simulink model "SimulinkBATproject"  (R2022b)
settings: Solver=FixedStepAuto  StartTime=0.0  StopTime=15  FixedStep=1e-4  RelTol=1e-3
libraries: spsDiodeLib x12, spsPVArrayLib x10, spsSeriesRLCBranchLib x5, spsCurrentMeasurementLib x1, spsMosfetLib x1, spsPWMGeneratorDCDCLib x1, spsVoltageMeasurementLib x1, spspowerguiLib x1
settings Model: Creator=ACER  LastModifiedBy=LE QUOC DINH
settings SolverCC: AlgebraicLoopSolver=TrustRegion
settings DataIOCC: ReturnWorkspaceOutputs=off
settings DebuggingCC: UnconnectedInputMsg=warning  UnconnectedOutputMsg=warning  UnconnectedLineMsg=warning  PregeneratedLibrarySubsystemCodeDiagnostic=none  SFMachineParentedDataDiag=warning  ArithmeticOperatorsInVariantConditions=warning
settings ModelReferenceCC: EnableRefExpFcnMdlSchedulingChecks=on
settings SFSimCC: SimUseLocalCustomCode=off  CustomCodeUndefinedFunction=UseInterfaceOnly
settings RTWCC: RTWUseLocalCustomCode=off

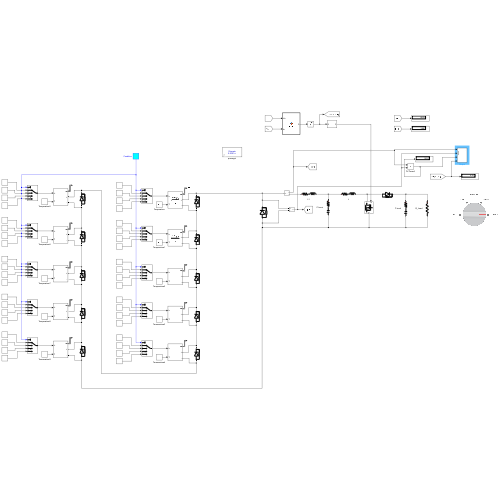
[thumbnail: Simulink's stored preview of the top-level diagram]
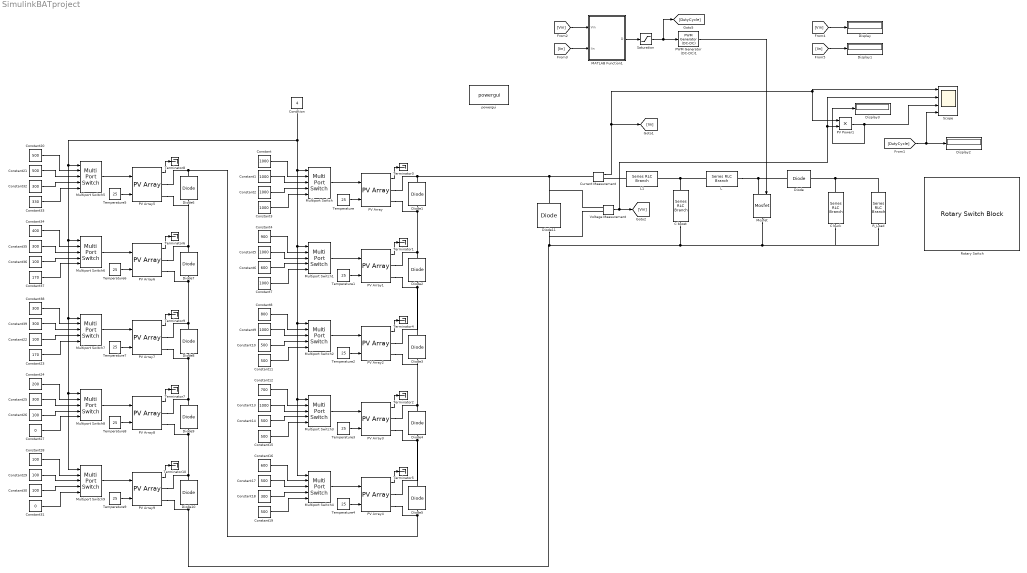
== system SimulinkBATproject ==
  C boost : spsSeriesRLCBranchLib/Series RLC Branch  LConnTagsString=__new0  RConnTagsString=__new0  BranchType=RC  Resistance=1  Inductance=1e-3  SetiL0=off  InitialCurrent=0  Capacitance=50e-3  Setx0=off  InitialVoltage=0  Measurements=None
  C buck : spsSeriesRLCBranchLib/Series RLC Branch  LConnTagsString=__new0  RConnTagsString=__new0  BranchType=RC  Resistance=1  Inductance=1e-3  SetiL0=off  InitialCurrent=0  Capacitance=150e-6  Setx0=off  InitialVoltage=0  Measurements=None
  Condition : Constant  Value=4
  Constant{,1..3,5,7,9,13} (8 alike) : Constant  Value=1000
  Constant{10..11,14..15,17,19..21} (8 alike) : Constant  Value=500
  Constant12 : Constant  Value=700
  Constant16 : Constant  Value=600
  Constant{18,25,32,35,38..39} (6 alike) : Constant  Value=300
  Constant{22,26,28..30,36} (6 alike) : Constant  Value=100
  Constant23 : Constant  Value=170
  Constant24 : Constant  Value=200
  Constant27 : Constant  Value=0
  Constant31 : Constant  Value=0
  Constant33 : Constant  Value=330
  Constant34 : Constant  Value=400
  Constant37 : Constant  Value=170
  Constant4 : Constant  Value=900
  Constant6 : Constant  Value=600
  Constant8 : Constant  Value=800
  Current Measurement : spsCurrentMeasurementLib/Current Measurement  PhasorSimulation=off  OutputType=Complex  PSBequivalent=0
  Diode{,1..11} (12 alike) : spsDiodeLib/Diode  Ron=0.001  Lon=0  Vf=0.8  IC=0  UseSnubber=0  Rs=500  Cs=250e-9  Measurements=off
  Display{,1..3} (4 alike) : Display
  L : spsSeriesRLCBranchLib/Series RLC Branch  LConnTagsString=__new0  RConnTagsString=__new0  BranchType=RL  Resistance=1  Inductance=100e-3  SetiL0=off  InitialCurrent=0  Capacitance=1e-6  Setx0=off  InitialVoltage=0  Measurements=None
  L1 : spsSeriesRLCBranchLib/Series RLC Branch  LConnTagsString=__new0  RConnTagsString=__new0  BranchType=RL  Resistance=1  Inductance=100e-3  SetiL0=off  InitialCurrent=0  Capacitance=1e-6  Setx0=off  InitialVoltage=0  Measurements=None
  MATLAB Function1 : MATLAB Function  TreatAsAtomicUnit=on
  Mosfet : spsMosfetLib/Mosfet  Ron=0.1  Lon=0  Rd=0.01  Vfd=0  IC=0  Rs=1e5  Cs=inf  Measurements=off
  Multiport Switch{,1..9} (10 alike) : MultiPortSwitch  Inputs=4  SaturateOnIntegerOverflow=off  InputSameDT=off
  PV Array{,1..9} (10 alike) : spsPVArrayLib/PV Array  Npar=1  Nser=1  PlotType=array @ 25 deg.C & specified irradiances  S_vec="[ 1000  500  100 ]"  Temp_C_vec="[ 45 25  ]"  ModuleName=Mitsubishi Electric PV-EE125MF5F  PlotWhenSelected=off  Pm=125.079  Ncell=36  Voc=21.8  Isc=7.9  Vm=17.3  Im=7.23  beta_Voc_pc=-0.3637  alpha_Isc_pc=0.042696  beta_Voc=-0.079287  alpha_Isc=0.003373  IL=7.9305  I0=2.9341e-10  nI=0.98298  Rsh=66.3188  Rs=0.25575  RobustModel=off  RobustCellTemperature=313.3991  BAL=off  Tc=20  Tfilter=0.1
  PV Power1 : Product
  PWM Generator (DC-DC)1 : spsPWMGeneratorDCDCLib/PWM Generator (DC-DC)  Fsw=5000  Ts=0
  R_Load : spsSeriesRLCBranchLib/Series RLC Branch  LConnTagsString=__new0  RConnTagsString=__new0  BranchType=R  Resistance=90.2  Inductance=50e-6  SetiL0=off  InitialCurrent=0  Capacitance=1000e-6  Setx0=off  InitialVoltage=0  Measurements=None
  Rotary Switch : RotarySwitchBlock
      settings: Values={{'Condition A', 'Condition B', 'Condition C', 'Condition D'}, [1 2 3 4]}
  Saturation : Saturate  UpperLimit=1  LowerLimit=0
  Scope : Scope  NumInputPorts=4
  Temperature{,1..9} (10 alike) : Constant  Value=25
  Terminator{1..10} (10 alike) : Terminator
  Voltage Measurement : spsVoltageMeasurementLib/Voltage Measurement  PhasorSimulation=off  OutputType=Complex  PSBequivalent=0
  powergui : spspowerguiLib/powergui  Priority=1  SimulationMode=Discrete  SampleTime=1e-4  frequency=60  Iterations=50  frequencyindice=0  Pbase=100e6  ErrMax=1e-4  UnitsV=kV  UnitsW=MW  buscounter=0  FunctionMessages=off  echomessages=off  EnableUseOfTLC=off  CurrentSourceSwitches=off  DisableSnubberDevices=off  DisableRonSwitches=off  DisableVfSwitches=off  DisplayEquations=off  AutomaticDiscreteSolvers=off  SolverType=Tustin  Interpol=off  ExternalGateDelay=off  methode=off  Ts=100  x0status=blocks  SPID=on  SwTol=0  HookPort=off  NonlinearTolerance=1e-4  nMaxIteration=100  ContinueOnMaxIteration=off  RestoreLinks=warning  ResistiveCurrentMeasurement=off  Frange=[0:2:500]  Ylog=off  Xlog=on  ShowGrid=off  save=off  variable=ZData  structure=0  ZoomFFT=off  StartTime=0.0  cycles=1  DisplayStyle=1  fundamental=60  FreqAxis=off  MaxFrequency=1000  frequencyindicesteady=1  RmsSteady=1  display=off
  wires:
  Current Measurement/1 -> PV Power1/1, Scope/1, [Iin]
  Voltage Measurement/1 -> [Vin], Scope/2, PV Power1/2
  PV Power1/1 -> Display3/1, Scope/3
  Multiport Switch1/1 -> PV Array1/1
  PV Array7/1 -> Terminator9/1
  Multiport Switch8/1 -> PV Array8/1
  Temperature8/1 -> PV Array8/2
  Constant39/1 -> Multiport Switch7/3
  Constant14/1 -> Multiport Switch3/4
  Constant21/1 -> Multiport Switch5/3
  Multiport Switch5/1 -> PV Array5/1
  PV Array6/1 -> Terminator6/1
  PV Array8/1 -> Terminator7/1
  Constant32/1 -> Multiport Switch5/4
  PV Array2/1 -> Terminator4/1
  Constant11/1 -> Multiport Switch2/5
  Constant33/1 -> Multiport Switch5/5
  Constant37/1 -> Multiport Switch6/5
  PV Array/1 -> Terminator3/1
  Constant6/1 -> Multiport Switch1/4
  Temperature4/1 -> PV Array4/2
  Temperature3/1 -> PV Array3/2
  Temperature7/1 -> PV Array7/2
  PV Array4/1 -> Terminator5/1
  Constant35/1 -> Multiport Switch6/3
  Constant36/1 -> Multiport Switch6/4
  Constant24/1 -> Multiport Switch8/2
  Constant26/1 -> Multiport Switch8/4
  Temperature6/1 -> PV Array6/2
  Constant31/1 -> Multiport Switch9/5
  Multiport Switch6/1 -> PV Array6/1
  Constant27/1 -> Multiport Switch8/5
  Constant34/1 -> Multiport Switch6/2
  Constant28/1 -> Multiport Switch9/2
  Constant19/1 -> Multiport Switch4/5
  Constant38/1 -> Multiport Switch7/2
  Multiport Switch7/1 -> PV Array7/1
  PV Array9/1 -> Terminator10/1
  Constant23/1 -> Multiport Switch7/5
  Constant30/1 -> Multiport Switch9/4
  Constant29/1 -> Multiport Switch9/3
  Multiport Switch9/1 -> PV Array9/1
  PV Array5/1 -> Terminator8/1
  Temperature9/1 -> PV Array9/2
  Multiport Switch4/1 -> PV Array4/1
  Constant18/1 -> Multiport Switch4/4
  Constant17/1 -> Multiport Switch4/3
  Constant8/1 -> Multiport Switch2/2
  Constant9/1 -> Multiport Switch2/3
  Temperature2/1 -> PV Array2/2
  Multiport Switch2/1 -> PV Array2/1
  Constant22/1 -> Multiport Switch7/4
  Constant10/1 -> Multiport Switch2/4
  PV Array1/1 -> Terminator1/1
  Constant12/1 -> Multiport Switch3/2
  Temperature5/1 -> PV Array5/2
  Constant4/1 -> Multiport Switch1/2
  Constant16/1 -> Multiport Switch4/2
  Constant7/1 -> Multiport Switch1/5
  Constant5/1 -> Multiport Switch1/3
  Constant3/1 -> Multiport Switch/5
  PV Array3/1 -> Terminator2/1
  Multiport Switch/1 -> PV Array/1
  Constant20/1 -> Multiport Switch5/2
  Constant2/1 -> Multiport Switch/4
  Constant1/1 -> Multiport Switch/3
  Constant13/1 -> Multiport Switch3/3
  Temperature1/1 -> PV Array1/2
  Constant/1 -> Multiport Switch/2
  Multiport Switch3/1 -> PV Array3/1
  Constant15/1 -> Multiport Switch3/5
  Temperature/1 -> PV Array/2
  Constant25/1 -> Multiport Switch8/3
  Condition/1 -> Multiport Switch2/1, Multiport Switch4/1, Multiport Switch3/1, Multiport Switch1/1, Multiport Switch/1, Multiport Switch5/1, Multiport Switch6/1, Multiport Switch8/1, Multiport Switch9/1, Multiport Switch7/1
  [Iin] -> MATLAB Function1/2(Iin)
  MATLAB Function1/1(D) -> Saturation/1
  [Vin] -> MATLAB Function1/1(Vin)
  Saturation/1 -> [DutyCycle], PWM Generator (DC-DC)1/1
  PWM Generator (DC-DC)1/1 -> Mosfet/1
  [DutyCycle] -> Display2/1, Scope/4
  [Vin] -> Display/1
  [Iin] -> Display1/1
  connections:
  Diode1/RConn1 -- Voltage Measurement/LConn1 -- Diode11/RConn1 -- Current Measurement/LConn1 -- PV Array/RConn1
  Diode/LConn1 -- L/RConn1 -- Mosfet/LConn1
  PV Array9/RConn2 -- Voltage Measurement/LConn2 -- Diode11/LConn1 -- C boost/RConn1 -- Mosfet/RConn1 -- C buck/RConn1 -- R_Load/RConn1 -- Diode10/LConn1
  C buck/LConn1 -- R_Load/LConn1 -- Diode/RConn1
  C boost/LConn1 -- L1/RConn1 -- L/LConn1
  Diode6/RConn1 -- PV Array5/RConn1 -- PV Array4/RConn2 -- Diode5/LConn1
  PV Array7/RConn1 -- Diode8/RConn1 -- PV Array6/RConn2 -- Diode7/LConn1
  PV Array7/RConn2 -- Diode8/LConn1 -- Diode9/RConn1 -- PV Array8/RConn1
  PV Array9/RConn1 -- Diode10/RConn1 -- Diode9/LConn1 -- PV Array8/RConn2
  PV Array6/RConn1 -- Diode7/RConn1 -- PV Array5/RConn2 -- Diode6/LConn1
  Diode2/LConn1 -- PV Array2/RConn1 -- Diode3/RConn1 -- PV Array1/RConn2
  Diode1/LConn1 -- PV Array1/RConn1 -- Diode2/RConn1 -- PV Array/RConn2
  Diode4/RConn1 -- PV Array3/RConn1 -- PV Array2/RConn2 -- Diode3/LConn1
  PV Array3/RConn2 -- Diode5/RConn1 -- PV Array4/RConn1 -- Diode4/LConn1
  L1/LConn1 -- Current Measurement/RConn1

== matlab function SimulinkBATproject/MATLAB Function1 ==
  settings: updateMethod=DISCRETE
  data: Vin input; D output; Iin input
function D = BAT(Vin,Iin)

coder.extrinsic('randi')

persistent u;
persistent i;
persistent j;
persistent k;                  % Iterations
persistent DP;                 % DutyCycle   
persistent DPcurrent;          % Current DutyCycle      
persistent v;                  % Velocity
persistent F;                  % Frequency
persistent Fmax;               % Maximum frequency
persistent Fmin;               % Minimum frequency
persistent A;                  % Loudness
persistent r;                  % Pulse emission rate
persistent bestDP;
persistent DPcontainer;
persistent DPfitness;
persistent P;                  % Power
persistent Pfitness;
persistent counter;            % Counter
persistent lb;                 % Lower boundary
persistent ub;                 % Upper boundary
persistent ro;                 % Initial pulse emission rate
persistent alpha;              % Constant for loudness update
persistent gamma;              % Constant for emission rate update
persistent eps;
persistent Pprev; 
persistent bool; 
persistent closeness;
persistent index;

%initialization
if (isempty(counter))
    counter=0;
    bool=0;
    index=0;
    closeness=false;
    Pprev=Vin*Iin;
    k=0;                    % Iterations
    lb=0;                   % Lower boundary
    ub=1;                   % Upper boundary
    DPcurrent=0.5;          % Current DutyCycle  
    DPcontainer=zeros(4,1);
    DPfitness=zeros(4,1);
    Fmax=0.5;               % Maximum frequency
    Fmin=0.3;               % Minimum frequency
    A=rand(4,1);            % Loudness for each DutyCycle
    r=rand(4,1);            % Pulse emission rate for each DutyCycle
    u=0;
    i=0;
    v=zeros(4,1);           % Velocities
    F=zeros(4,1);           % Frequency
    P=zeros(4,1);           % Power
    Pfitness=zeros(4,1);
    alpha=0.5;              % Constant for loudness update
    gamma=0.5;              % Constant for emission rate update
    ro=0.67;                % Initial pulse emission rate
    DP=zeros(4,1);          % Dutycycles
    %initial dc for each particle
    DP(1)=0.2;
    DP(2)=0.4;
    DP(3)=0.6;
    DP(4)=0.8;       
end

% At the first time, this if ignored (counter=0)
% Delay
if(counter>=1 && counter<300)
    D=DPcurrent;
    counter=counter+1;
    return;              % return control to the invoking function before it reaches the end of the function.
end
counter=0;               % reset the counter

% calculate the fittnes function (power) of each particle
% then compare the current value of the function with the previous one
% if the current value is better than the previous, update the value
% Note: at the first time, this if ignored (u=0)
if(u>=1 && u<=4)
    P(u)=Vin*Iin;
    DPcontainer(u)=DPcurrent;    
end

% Update if the solution improves, or not too loud
if(u>4)
    for i=1:4
        if (P(i)>=Pfitness(i)) 
            Pfitness(i)=P(i);
            DPfitness(i)=DPcontainer(i);
            if(k>=1)  
                A(i)=alpha*A(i);
                r(i)=ro*(1-exp(-gamma*k));
            end
        end
    end
end

u=u+1;
% AT the first time, this is excuted because it consist the condition...
% u==0 (initial value of u)
if(u==6)
    u=1;
end

if(u==5)
    if(bool==0)
        k=k+1;    
    end

    [Pmax,index]=max(Pfitness);            % finds the indices of the maximum values of P (max power) and returns them in output vector "index"
    bestDP=DPfitness(index);               % find the location(duty) of the particle which has max Power
    if(bool==0)
        D=bestDP;
    else
        D=DP(index);         %mean          
    end
    DPcurrent=D;
    counter=1;

    for i=1:4
        F(i)=Fmin+(Fmax-Fmin)*rand;                     %randomly chose the frequency
        v(i)=v(i)+(DPfitness(i)-bestDP)*F(i);           %update the velocity
        if DPfitness(i)>bestDP
            DP(i)=DPfitness(i)-abs(v(i));               %update the Dutycycle position
        else
            DP(i)=DPfitness(i)+abs(v(i));               %update the Dutycycle position
        end
 
        %Checking bounds/limits
        if DP(i) < lb % Check the lower limit
            DP(i) = lb;
        elseif DP(i) > ub % Check the upper limit
            DP(i) = ub;
        end

        %check the condition with r
        if rand>r(i)
            eps=-1+(1-(-1))*rand;
            DP(i)=bestDP+eps*mean(A);
        end        
    end

    if(bool==0)
        closeness=true;
        for i=1:4
            for j=1:4
                if(i~=j)
                    closeness = closeness & (abs(DP(i)-DP(j))<0.1);       %0.05
                end
            end
        end
    end

    %if the power stables already
    if(bool==1 )        
        %check if the power changes
        if(abs(Vin*Iin-Pprev)/Pprev >= 0.05)           %0.1
            
            DPcurrent=0.5;          % Current DutyCycle  
            DPcontainer=zeros(4,1);
            DPfitness=zeros(4,1);
            A=rand(4,1);            % Loudness for each DutyCycle
            r=rand(4,1);            % Pulse emission rate for each DutyCycle
            v=zeros(4,1);           % Velocities
            F=zeros(4,1);           % Frequency
            P=zeros(4,1);           % Power
            Pfitness=zeros(4,1);
            DP=zeros(4,1);          % Dutycycles
               
            DP(1)=randi([5 250])/1000;
            DP(2)=randi([250 500])/1000;
            DP(3)=randi([500 750])/1000;
            DP(4)=randi([760 995])/1000;
                
            bool=0;           
        end     
    end
        
    if(closeness==1)
        bool=1; 
        closeness=false;   
    end
    
    if(k>100)
          
            DPcurrent=0.5;          % Current DutyCycle  
            DPcontainer=zeros(4,1);
            DPfitness=zeros(4,1);
            A=rand(4,1);            % Loudness for each DutyCycle
            r=rand(4,1);            % Pulse emission rate for each DutyCycle
            v=zeros(4,1);           % Velocities
            F=zeros(4,1);           % Frequency
            P=zeros(4,1);           % Power
            Pfitness=zeros(4,1);
            DP=zeros(4,1);          % Dutycycles
               
            DP(1)=randi([5 250])/1000;
            DP(2)=randi([250 500])/1000;
            DP(3)=randi([500 750])/1000;
            DP(4)=randi([760 995])/1000;
                
            k=0;
    end
        
    Pprev = Vin*Iin;

    return;
else
    %update each particle's duty cycle, reset counter. 
    if(bool==0)
        D=DP(u);
    else
        D=DP(index); %mean          
    end
    DPcurrent=D;
    return; 
end    
end
